simulink model "Final2023"  (R2016a)
settings: Solver=VariableStepAuto  StartTime=0.0  StopTime=10.0  RelTol=1e-3
libraries: visiontextngfix x1, simulink x1
settings Model: Creator=alber  LastModifiedBy=alber

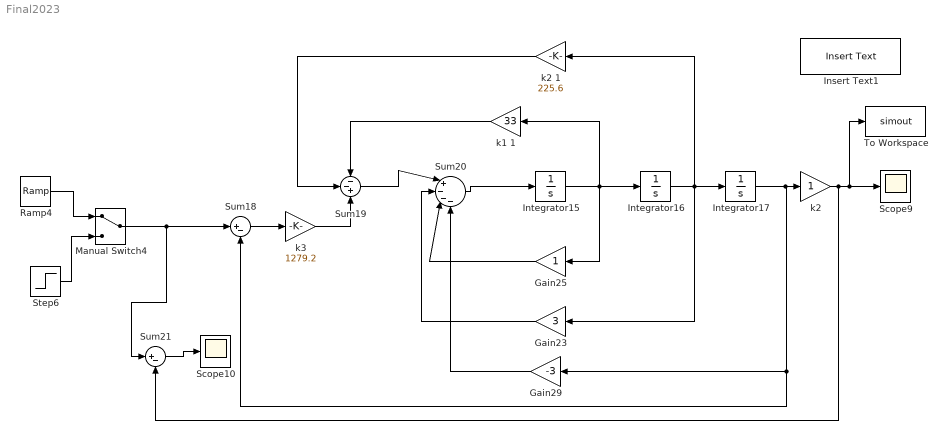
== system Final2023 ==
  Gain23 : Gain  Gain=3
  Gain25 : Gain
  Gain29 : Gain  Gain=-3
  Insert Text1 : visiontextngfix/Insert Text  inputType=Obsolete  theText='Febrero_23'  getTextLocFrom=Specify via dialog  textLoc=[1 1]  getTextColorFrom=Specify via dialog  textColor=[0 0 0]  getTextIntensityFrom=Specify via dialog  textIntensity=0  getTextOpacityFrom=Specify via dialog  textOpacity=1.0  dummyVar2=0  dummyVar3=0  dummyVar4=0  imagePorts=One multidimensional signal  isInputTransposed=off  fontFace=LucidaSansRegular  dummyVar1=0  blockFontSize=12  antiAliased=on
  Integrator15 : Integrator
  Integrator16 : Integrator
  Integrator17 : Integrator
  Manual Switch4 : ManualSwitch
  Ramp4 : simulink/Sources/Ramp  slope=1  start=0  X0=0
  Scope10 : Scope
  Scope9 : Scope
  Step6 : Step  Time=0  SampleTime=0
  Sum18 : Sum  Inputs=|+-
  Sum19 : Sum  Inputs=--+
  Sum20 : Sum  Inputs=|+---
  Sum21 : Sum  Inputs=|+-
  To Workspace : ToWorkspace  VariableName=simout  SaveFormat=Timeseries  SampleTime=-1
  k1 1 : Gain  Gain=33
  k2 : Gain
  k2 1 : Gain  Gain=225.6
  k3 : Gain  Gain=1279.2
  wires:
  Ramp4/1 -> Manual Switch4/1
  Step6/1 -> Manual Switch4/2
  Manual Switch4/1 -> Sum21/1, Sum18/1
  Integrator15/1 -> k1 1/1, Gain25/1, Integrator16/1
  Sum20/1 -> Integrator15/1
  Gain25/1 -> Sum20/3
  Gain23/1 -> Sum20/2
  Integrator16/1 -> Integrator17/1, k2 1/1, Gain23/1
  Sum19/1 -> Sum20/1
  k1 1/1 -> Sum19/1
  Sum18/1 -> k3/1
  Sum21/1 -> Scope10/1
  k2 1/1 -> Sum19/2
  k3/1 -> Sum19/3
  Integrator17/1 -> Sum18/2, Gain29/1, k2/1
  Gain29/1 -> Sum20/4
  k2/1 -> Sum21/2, To Workspace/1, Scope9/1
